simulink model "Attitude_Control_Model_ECX_Flat22L_4Axis"  (R2024b)
settings: Solver=VariableStepAuto  StartTime=0.0  StopTime=10.0  RelTol=1e-3
libraries: slpidlib x7, simulink_extras x2, aerolibutil x2, matrix_library x1
settings Model: Creator=LEGION  LastModifiedBy=LEGION

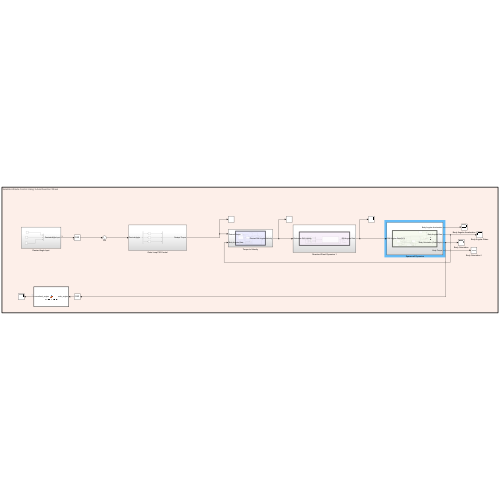
[thumbnail: Simulink's stored preview of the top-level diagram]
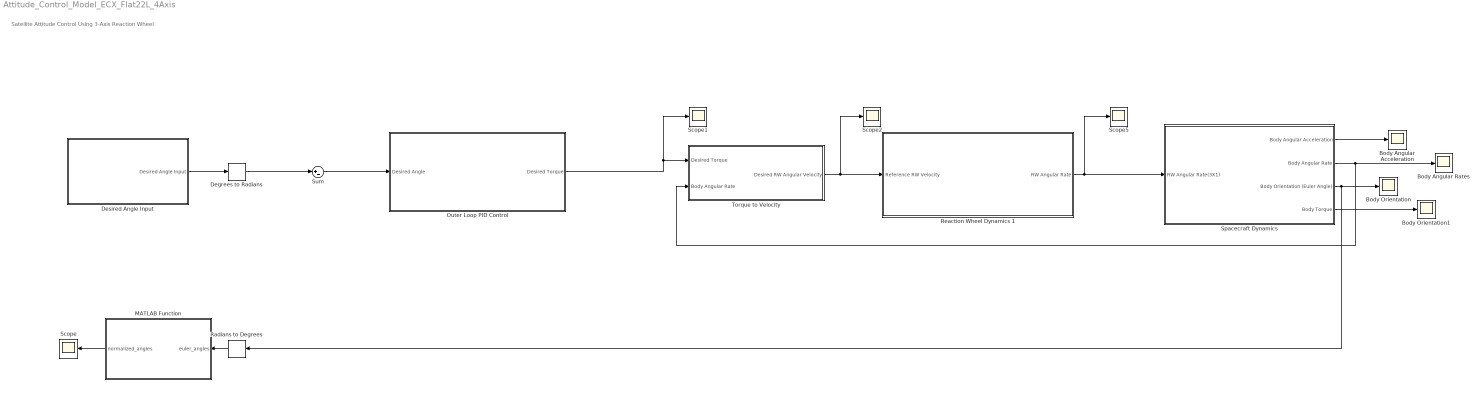
== system Attitude_Control_Model_ECX_Flat22L_4Axis ==
  note: Satellite Attitude Control Using 3-Axis Reaction Wheel
  Body Angular Acceleration : Scope
  Body Angular Rates : Scope
  Body Orientation : Scope
  Body Orientation1 : Scope
  Degrees to Radians : simulink_extras/Transformations/Degrees to Radians
  Desired Angle Input : Subsystem
  MATLAB Function : MATLAB Function  TreatAsAtomicUnit=on
  Outer Loop PID Control : Subsystem
  Radians to Degrees : simulink_extras/Transformations/Radians to Degrees
  Reaction Wheel Dynamics 1 : Subsystem
  Scope{,1..2,5} (4 alike) : Scope
  Spacecraft Dynamics : Subsystem
  Sum : Sum  Inputs=|+-
  Torque to Velocity : Subsystem
  wires:
  Outer Loop PID Control/1(Desired Torque) -> Scope1/1, Torque to Velocity/1(Desired Torque)
  Sum/1 -> Outer Loop PID Control/1(Desired Angle)
  Degrees to Radians/1 -> Sum/1
  Desired Angle Input/1(Desired Angle Input) -> Degrees to Radians/1
  Reaction Wheel Dynamics 1/1(RW Angular Rate) -> Spacecraft Dynamics/1(RW Angular Rate(3X1)), Scope5/1
  Radians to Degrees/1 -> MATLAB Function/1(euler_angles)
  Torque to Velocity/1(Desired RW Angular Velocity) -> Reaction Wheel Dynamics 1/1(Reference RW Velocity), Scope2/1
  MATLAB Function/1(normalized_angles) -> Scope/1
  Spacecraft Dynamics/1(Body Angular Acceleration) -> Body Angular Acceleration/1
  Spacecraft Dynamics/2(Body Angular Rate) -> Torque to Velocity/2(Body Angular Rate), Body Angular Rates/1
  Spacecraft Dynamics/3(Body Orientation (Euler Angle)) -> Radians to Degrees/1, Body Orientation/1
  Spacecraft Dynamics/4(Body Torque) -> Body Orientation1/1

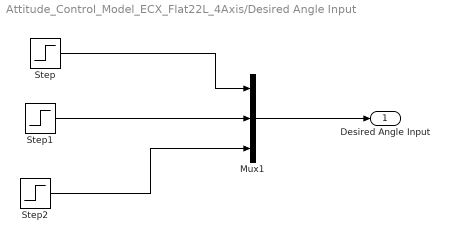
== system Attitude_Control_Model_ECX_Flat22L_4Axis/Desired Angle Input ==
  Mux1 : Mux  Inputs=3
  Step : Step  Time=0.1  After=270  SampleTime=0  VectorParams1D=off
  Step1 : Step  Time=0.1  After=90  SampleTime=0  VectorParams1D=off
  Step2 : Step  Time=0.1  After=90  SampleTime=0  VectorParams1D=off
  Desired Angle Input : Outport
  wires:
  Mux1/1 -> Desired Angle Input/1
  Step1/1 -> Mux1/2
  Step/1 -> Mux1/1
  Step2/1 -> Mux1/3

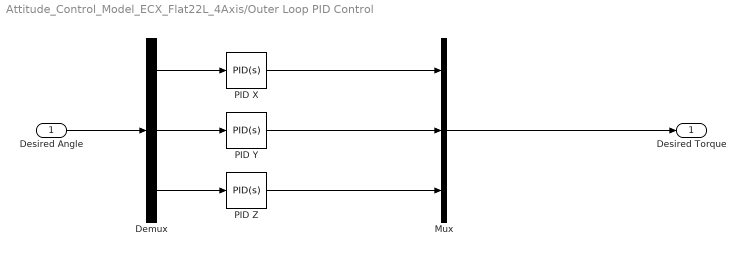
== system Attitude_Control_Model_ECX_Flat22L_4Axis/Outer Loop PID Control ==
  Desired Angle : Inport
  Demux : Demux  Outputs=3
  Mux : Mux  Inputs=3
  PID X : slpidlib/PID Controller  Controller=PID  Form=Parallel  TimeDomain=Continuous-time  UseExternalTs=off  SampleTime=-1  IntegratorMethod=Forward Euler  FilterMethod=Forward Euler  ControllerParametersSource=internal  P=0.8  I=0.007  UseKiTs=off  D=0.5  UseExternalDerivativeSource=off  N=100  UseFilter=on  TunerSelectOption=Transfer Function Based (PID Tuner App)  InitialConditionSource=internal  InitialConditionForIntegrator=0  InitialConditionForFilter=0  DifferentiatorICPrevScaledInput=0  ExternalReset=none  TrackingMode=off  Kt=1  LimitOutput=off  SatLimitsSource=internal  UpperSaturationLimit=inf  LowerSaturationLimit=-inf  LinearizeAsGain=on  AntiWindupMode=none  Kb=1  LimitIntegrator=off  UpperIntegratorSaturationLimit=inf  LowerIntegratorSaturationLimit=-inf  POutMin=[]  POutMax=[]  IOutMin=[]  IOutMax=[]  DOutMin=[]  DOutMax=[]  NOutMin=[]  NOutMax=[]  SumOutMin=[]  SumOutMax=[]  SaturationOutMin=[]  SaturationOutMax=[]  PParamMin=[]  PParamMax=[]  IParamMin=[]  IParamMax=[]  DParamMin=[]  DParamMax=[]  NParamMin=[]  NParamMax=[]  KbParamMin=[]  KbParamMax=[]  KtParamMin=[]  KtParamMax=[]  KbOutMin=[]  KbOutMax=[]  KtOutMin=[]  KtOutMax=[]  IntegratorOutMin=[]  IntegratorOutMax=[]  FilterOutMin=[]  FilterOutMax=[]  SumI1OutMin=[]  SumI1OutMax=[]  SumI2OutMin=[]  SumI2OutMax=[]  SumI3OutMin=[]  SumI3OutMax=[]  SumI4OutMin=[]  SumI4OutMax=[]  SumDOutMin=[]  SumDOutMax=[]  DifferentiatorOutMin=[]  DifferentiatorOutMax=[]  FilterDiffOutCoefMin=[]  FilterDiffOutCoefMax=[]  ReciprocalOutMin=[]  ReciprocalOutMax=[]  SumDenOutMin=[]  SumDenOutMax=[]  SumNumOutMin=[]  SumNumOutMax=[]  DivideOutMin=[]  DivideOutMax=[]  UdiffTsProdOutMin=[]  UdiffTsProdOutMax=[]  NTsProdOutMin=[]  NTsProdOutMax=[]  UintegralTsProdOutMin=[]  UintegralTsProdOutMax=[]  UngainTsProdOutMin=[]  UngainTsProdOutMax=[]  ClampingZeroOutDataTypeStr=Inherit: Inherit via back propagation  ClampingZeroOutMin=[]  ClampingZeroOutMax=[]  FilterDenConstantOutDataTypeStr=Inherit: Inherit via back propagation  FilterDenConstantOutMin=[]  FilterDenConstantOutMax=[]  PCopyOutDataTypeStr=Inherit: Inherit via back propagation  PCopyOutMin=[]  PCopyOutMax=[]  NCopyOutDataTypeStr=Inherit: Inherit via back propagation  NCopyOutMin=[]  NCopyOutMax=[]  IntegratorContinuousStateAttributes=''  IntegratorStateMustResolveToSignalObject=off  IntegratorRTWStateStorageClass=Auto  FilterContinuousStateAttributes=''  FilterStateMustResolveToSignalObject=off  FilterRTWStateStorageClass=Auto  ParallelPVariant=InternalParameters  IdealPVariant=Disabled  IVariant=InternalParameters  DVariant=InternalParameters  IntegratorVariant=Continuous  SatVariant=Disabled  AWVariant=Passthrough  PCopyVariant=Disabled  TRVariant=Disabled  FdbkBlocksVariant=Forward  IdealPFdbkVariant=Disabled  SatFdbkVariant=Disabled  DerivativeFilterVariant=ContFilter  NVariant=InternalParameters  NCopyVariant=Disabled  FilterICVariant=InternalICsFilter  IntegratorICVariant=InternalICs  ExternalResetVariant=Disabled  TRSumVariant=Passthrough  SumFdbkVariant=Disabled  SumVariant=Sum_PID  TsampFilterVariant=InternalTs  TsampNgainVariant=Passthrough  TsampIntegralVariant=Disabled_SignalSpec  ExternalSaturationOutDataTypeStr=Inherit: Same as second input  DerivativeSourceVariant=ErrorSignal  PreIntVariant=InternalPreInt
  PID Y : slpidlib/PID Controller  Controller=PID  Form=Parallel  TimeDomain=Continuous-time  UseExternalTs=off  SampleTime=-1  IntegratorMethod=Forward Euler  FilterMethod=Forward Euler  ControllerParametersSource=internal  P=0.5  I=0.06  UseKiTs=off  D=0.1  UseExternalDerivativeSource=off  N=100  UseFilter=on  TunerSelectOption=Transfer Function Based (PID Tuner App)  InitialConditionSource=internal  InitialConditionForIntegrator=0  InitialConditionForFilter=0  DifferentiatorICPrevScaledInput=0  ExternalReset=none  TrackingMode=off  Kt=1  LimitOutput=off  SatLimitsSource=internal  UpperSaturationLimit=inf  LowerSaturationLimit=-inf  LinearizeAsGain=on  AntiWindupMode=none  Kb=1  LimitIntegrator=off  UpperIntegratorSaturationLimit=inf  LowerIntegratorSaturationLimit=-inf  POutMin=[]  POutMax=[]  IOutMin=[]  IOutMax=[]  DOutMin=[]  DOutMax=[]  NOutMin=[]  NOutMax=[]  SumOutMin=[]  SumOutMax=[]  SaturationOutMin=[]  SaturationOutMax=[]  PParamMin=[]  PParamMax=[]  IParamMin=[]  IParamMax=[]  DParamMin=[]  DParamMax=[]  NParamMin=[]  NParamMax=[]  KbParamMin=[]  KbParamMax=[]  KtParamMin=[]  KtParamMax=[]  KbOutMin=[]  KbOutMax=[]  KtOutMin=[]  KtOutMax=[]  IntegratorOutMin=[]  IntegratorOutMax=[]  FilterOutMin=[]  FilterOutMax=[]  SumI1OutMin=[]  SumI1OutMax=[]  SumI2OutMin=[]  SumI2OutMax=[]  SumI3OutMin=[]  SumI3OutMax=[]  SumI4OutMin=[]  SumI4OutMax=[]  SumDOutMin=[]  SumDOutMax=[]  DifferentiatorOutMin=[]  DifferentiatorOutMax=[]  FilterDiffOutCoefMin=[]  FilterDiffOutCoefMax=[]  ReciprocalOutMin=[]  ReciprocalOutMax=[]  SumDenOutMin=[]  SumDenOutMax=[]  SumNumOutMin=[]  SumNumOutMax=[]  DivideOutMin=[]  DivideOutMax=[]  UdiffTsProdOutMin=[]  UdiffTsProdOutMax=[]  NTsProdOutMin=[]  NTsProdOutMax=[]  UintegralTsProdOutMin=[]  UintegralTsProdOutMax=[]  UngainTsProdOutMin=[]  UngainTsProdOutMax=[]  ClampingZeroOutDataTypeStr=Inherit: Inherit via back propagation  ClampingZeroOutMin=[]  ClampingZeroOutMax=[]  FilterDenConstantOutDataTypeStr=Inherit: Inherit via back propagation  FilterDenConstantOutMin=[]  FilterDenConstantOutMax=[]  PCopyOutDataTypeStr=Inherit: Inherit via back propagation  PCopyOutMin=[]  PCopyOutMax=[]  NCopyOutDataTypeStr=Inherit: Inherit via back propagation  NCopyOutMin=[]  NCopyOutMax=[]  IntegratorContinuousStateAttributes=''  IntegratorStateMustResolveToSignalObject=off  IntegratorRTWStateStorageClass=Auto  FilterContinuousStateAttributes=''  FilterStateMustResolveToSignalObject=off  FilterRTWStateStorageClass=Auto  ParallelPVariant=InternalParameters  IdealPVariant=Disabled  IVariant=InternalParameters  DVariant=InternalParameters  IntegratorVariant=Continuous  SatVariant=Disabled  AWVariant=Passthrough  PCopyVariant=Disabled  TRVariant=Disabled  FdbkBlocksVariant=Forward  IdealPFdbkVariant=Disabled  SatFdbkVariant=Disabled  DerivativeFilterVariant=ContFilter  NVariant=InternalParameters  NCopyVariant=Disabled  FilterICVariant=InternalICsFilter  IntegratorICVariant=InternalICs  ExternalResetVariant=Disabled  TRSumVariant=Passthrough  SumFdbkVariant=Disabled  SumVariant=Sum_PID  TsampFilterVariant=InternalTs  TsampNgainVariant=Passthrough  TsampIntegralVariant=Disabled_SignalSpec  ExternalSaturationOutDataTypeStr=Inherit: Same as second input  DerivativeSourceVariant=ErrorSignal  PreIntVariant=InternalPreInt
  PID Z : slpidlib/PID Controller  Controller=PID  Form=Parallel  TimeDomain=Continuous-time  UseExternalTs=off  SampleTime=-1  IntegratorMethod=Forward Euler  FilterMethod=Forward Euler  ControllerParametersSource=internal  P=0.8  I=0.0005  UseKiTs=off  D=1.5  UseExternalDerivativeSource=off  N=100  UseFilter=on  TunerSelectOption=Transfer Function Based (PID Tuner App)  InitialConditionSource=internal  InitialConditionForIntegrator=0  InitialConditionForFilter=0  DifferentiatorICPrevScaledInput=0  ExternalReset=none  TrackingMode=off  Kt=1  LimitOutput=off  SatLimitsSource=internal  UpperSaturationLimit=inf  LowerSaturationLimit=-inf  LinearizeAsGain=on  AntiWindupMode=none  Kb=1  LimitIntegrator=off  UpperIntegratorSaturationLimit=inf  LowerIntegratorSaturationLimit=-inf  POutMin=[]  POutMax=[]  IOutMin=[]  IOutMax=[]  DOutMin=[]  DOutMax=[]  NOutMin=[]  NOutMax=[]  SumOutMin=[]  SumOutMax=[]  SaturationOutMin=[]  SaturationOutMax=[]  PParamMin=[]  PParamMax=[]  IParamMin=[]  IParamMax=[]  DParamMin=[]  DParamMax=[]  NParamMin=[]  NParamMax=[]  KbParamMin=[]  KbParamMax=[]  KtParamMin=[]  KtParamMax=[]  KbOutMin=[]  KbOutMax=[]  KtOutMin=[]  KtOutMax=[]  IntegratorOutMin=[]  IntegratorOutMax=[]  FilterOutMin=[]  FilterOutMax=[]  SumI1OutMin=[]  SumI1OutMax=[]  SumI2OutMin=[]  SumI2OutMax=[]  SumI3OutMin=[]  SumI3OutMax=[]  SumI4OutMin=[]  SumI4OutMax=[]  SumDOutMin=[]  SumDOutMax=[]  DifferentiatorOutMin=[]  DifferentiatorOutMax=[]  FilterDiffOutCoefMin=[]  FilterDiffOutCoefMax=[]  ReciprocalOutMin=[]  ReciprocalOutMax=[]  SumDenOutMin=[]  SumDenOutMax=[]  SumNumOutMin=[]  SumNumOutMax=[]  DivideOutMin=[]  DivideOutMax=[]  UdiffTsProdOutMin=[]  UdiffTsProdOutMax=[]  NTsProdOutMin=[]  NTsProdOutMax=[]  UintegralTsProdOutMin=[]  UintegralTsProdOutMax=[]  UngainTsProdOutMin=[]  UngainTsProdOutMax=[]  ClampingZeroOutDataTypeStr=Inherit: Inherit via back propagation  ClampingZeroOutMin=[]  ClampingZeroOutMax=[]  FilterDenConstantOutDataTypeStr=Inherit: Inherit via back propagation  FilterDenConstantOutMin=[]  FilterDenConstantOutMax=[]  PCopyOutDataTypeStr=Inherit: Inherit via back propagation  PCopyOutMin=[]  PCopyOutMax=[]  NCopyOutDataTypeStr=Inherit: Inherit via back propagation  NCopyOutMin=[]  NCopyOutMax=[]  IntegratorContinuousStateAttributes=''  IntegratorStateMustResolveToSignalObject=off  IntegratorRTWStateStorageClass=Auto  FilterContinuousStateAttributes=''  FilterStateMustResolveToSignalObject=off  FilterRTWStateStorageClass=Auto  ParallelPVariant=InternalParameters  IdealPVariant=Disabled  IVariant=InternalParameters  DVariant=InternalParameters  IntegratorVariant=Continuous  SatVariant=Disabled  AWVariant=Passthrough  PCopyVariant=Disabled  TRVariant=Disabled  FdbkBlocksVariant=Forward  IdealPFdbkVariant=Disabled  SatFdbkVariant=Disabled  DerivativeFilterVariant=ContFilter  NVariant=InternalParameters  NCopyVariant=Disabled  FilterICVariant=InternalICsFilter  IntegratorICVariant=InternalICs  ExternalResetVariant=Disabled  TRSumVariant=Passthrough  SumFdbkVariant=Disabled  SumVariant=Sum_PID  TsampFilterVariant=InternalTs  TsampNgainVariant=Passthrough  TsampIntegralVariant=Disabled_SignalSpec  ExternalSaturationOutDataTypeStr=Inherit: Same as second input  DerivativeSourceVariant=ErrorSignal  PreIntVariant=InternalPreInt
  Desired Torque : Outport
  wires:
  PID X/1 -> Mux/1
  Demux/1 -> PID X/1
  PID Z/1 -> Mux/3
  Mux/1 -> Desired Torque/1
  Demux/2 -> PID Y/1
  Demux/3 -> PID Z/1
  PID Y/1 -> Mux/2
  Desired Angle/1 -> Demux/1

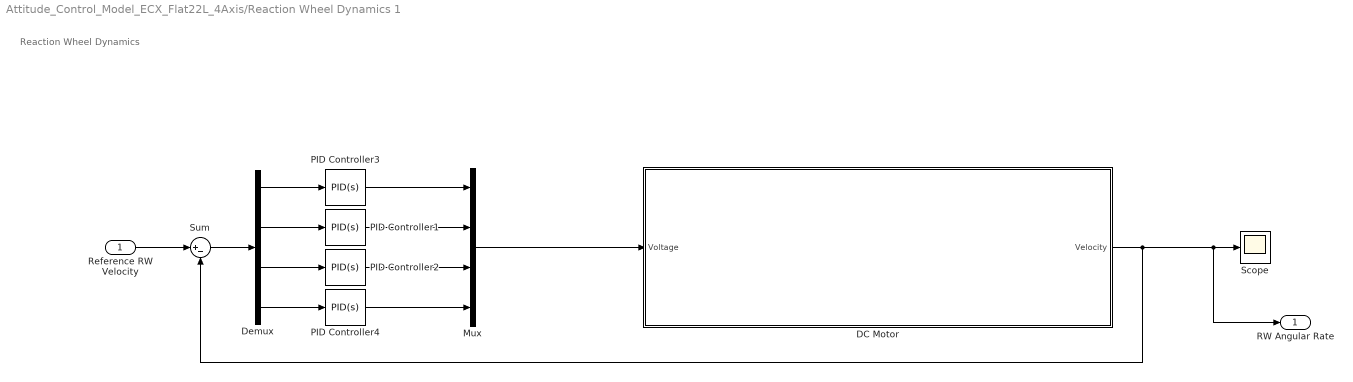
== system Attitude_Control_Model_ECX_Flat22L_4Axis/Reaction Wheel Dynamics 1 ==
  note: Reaction Wheel Dynamics
  Reference RW Velocity : Inport
  "DC Motor " : Subsystem
  Demux : Demux
  Mux : Mux
  PID Controller{1..4} (4 alike) : slpidlib/PID Controller  Controller=PID  Form=Parallel  TimeDomain=Continuous-time  UseExternalTs=off  SampleTime=-1  IntegratorMethod=Forward Euler  FilterMethod=Forward Euler  ControllerParametersSource=internal  P=0.5  I=0.005  UseKiTs=off  D=0.08  UseExternalDerivativeSource=off  N=100  UseFilter=on  TunerSelectOption=Transfer Function Based (PID Tuner App)  InitialConditionSource=internal  InitialConditionForIntegrator=0  InitialConditionForFilter=0  DifferentiatorICPrevScaledInput=0  ExternalReset=none  TrackingMode=off  Kt=1  LimitOutput=off  SatLimitsSource=internal  UpperSaturationLimit=inf  LowerSaturationLimit=-inf  LinearizeAsGain=on  AntiWindupMode=none  Kb=1  LimitIntegrator=off  UpperIntegratorSaturationLimit=inf  LowerIntegratorSaturationLimit=-inf  POutMin=[]  POutMax=[]  IOutMin=[]  IOutMax=[]  DOutMin=[]  DOutMax=[]  NOutMin=[]  NOutMax=[]  SumOutMin=[]  SumOutMax=[]  SaturationOutMin=[]  SaturationOutMax=[]  PParamMin=[]  PParamMax=[]  IParamMin=[]  IParamMax=[]  DParamMin=[]  DParamMax=[]  NParamMin=[]  NParamMax=[]  KbParamMin=[]  KbParamMax=[]  KtParamMin=[]  KtParamMax=[]  KbOutMin=[]  KbOutMax=[]  KtOutMin=[]  KtOutMax=[]  IntegratorOutMin=[]  IntegratorOutMax=[]  FilterOutMin=[]  FilterOutMax=[]  SumI1OutMin=[]  SumI1OutMax=[]  SumI2OutMin=[]  SumI2OutMax=[]  SumI3OutMin=[]  SumI3OutMax=[]  SumI4OutMin=[]  SumI4OutMax=[]  SumDOutMin=[]  SumDOutMax=[]  DifferentiatorOutMin=[]  DifferentiatorOutMax=[]  FilterDiffOutCoefMin=[]  FilterDiffOutCoefMax=[]  ReciprocalOutMin=[]  ReciprocalOutMax=[]  SumDenOutMin=[]  SumDenOutMax=[]  SumNumOutMin=[]  SumNumOutMax=[]  DivideOutMin=[]  DivideOutMax=[]  UdiffTsProdOutMin=[]  UdiffTsProdOutMax=[]  NTsProdOutMin=[]  NTsProdOutMax=[]  UintegralTsProdOutMin=[]  UintegralTsProdOutMax=[]  UngainTsProdOutMin=[]  UngainTsProdOutMax=[]  ClampingZeroOutDataTypeStr=Inherit: Inherit via back propagation  ClampingZeroOutMin=[]  ClampingZeroOutMax=[]  FilterDenConstantOutDataTypeStr=Inherit: Inherit via back propagation  FilterDenConstantOutMin=[]  FilterDenConstantOutMax=[]  PCopyOutDataTypeStr=Inherit: Inherit via back propagation  PCopyOutMin=[]  PCopyOutMax=[]  NCopyOutDataTypeStr=Inherit: Inherit via back propagation  NCopyOutMin=[]  NCopyOutMax=[]  IntegratorContinuousStateAttributes=''  IntegratorStateMustResolveToSignalObject=off  IntegratorRTWStateStorageClass=Auto  FilterContinuousStateAttributes=''  FilterStateMustResolveToSignalObject=off  FilterRTWStateStorageClass=Auto  ParallelPVariant=InternalParameters  IdealPVariant=Disabled  IVariant=InternalParameters  DVariant=InternalParameters  IntegratorVariant=Continuous  SatVariant=Disabled  AWVariant=Passthrough  PCopyVariant=Disabled  TRVariant=Disabled  FdbkBlocksVariant=Forward  IdealPFdbkVariant=Disabled  SatFdbkVariant=Disabled  DerivativeFilterVariant=ContFilter  NVariant=InternalParameters  NCopyVariant=Disabled  FilterICVariant=InternalICsFilter  IntegratorICVariant=InternalICs  ExternalResetVariant=Disabled  TRSumVariant=Passthrough  SumFdbkVariant=Disabled  SumVariant=Sum_PID  TsampFilterVariant=InternalTs  TsampNgainVariant=Passthrough  TsampIntegralVariant=Disabled_SignalSpec  ExternalSaturationOutDataTypeStr=Inherit: Same as second input  DerivativeSourceVariant=ErrorSignal  PreIntVariant=InternalPreInt
  Scope : Scope
  Sum : Sum  Inputs=|+-
  RW Angular Rate : Outport
  wires:
  "DC Motor "/1(Velocity) -> Sum/2, RW Angular Rate/1, Scope/1
  PID Controller1/1 -> Mux/2
  Demux/2 -> PID Controller1/1
  Demux/1 -> PID Controller3/1
  Demux/3 -> PID Controller2/1
  PID Controller3/1 -> Mux/1
  PID Controller2/1 -> Mux/3
  Mux/1 -> "DC Motor "/1(Voltage)
  Reference RW Velocity/1 -> Sum/1
  Sum/1 -> Demux/1
  Demux/4 -> PID Controller4/1
  PID Controller4/1 -> Mux/4

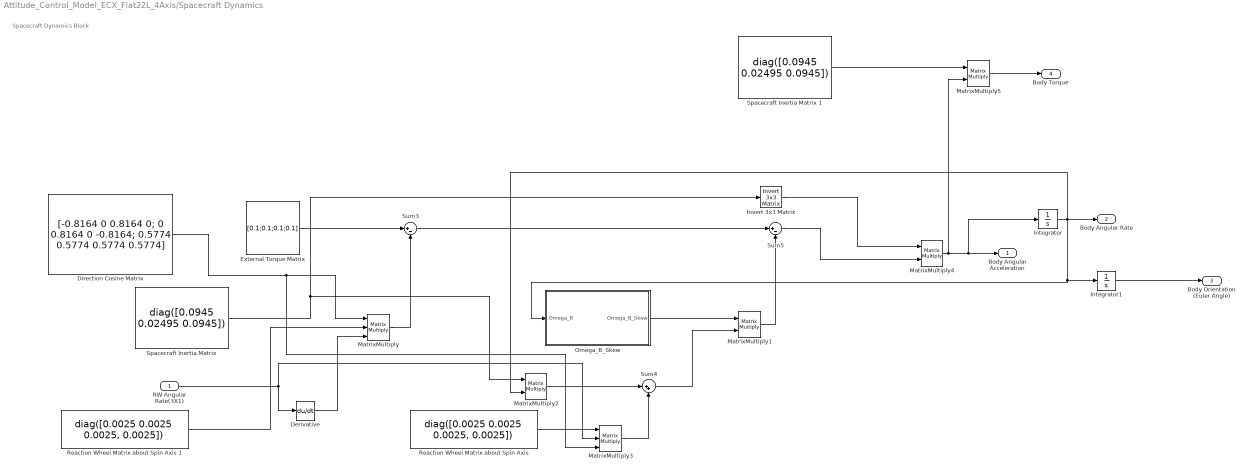
== system Attitude_Control_Model_ECX_Flat22L_4Axis/Spacecraft Dynamics ==
  note: Spacecraft Dynamics Block
  RW Angular Rate(3X1) : Inport
  Derivative : Derivative
  Direction Cosine Matrix : Constant  Value=[-0.8164 0 0.8164 0; 0 0.8164 0 -0.8164; 0.5774 0.5774 0.5774 0.5774]  VectorParams1D=off
  External Torque Matrix : Constant  Value=[0.1;0.1;0.1;0.1]  VectorParams1D=off
  Integrator : Integrator
  Integrator1 : Integrator
  Invert 3x3 Matrix : aerolibutil/Invert  3x3 Matrix
  MatrixMultiply : Product  Inputs=3  Multiplication=Matrix(*)
  MatrixMultiply{1..2,4..5} (4 alike) : Product  Multiplication=Matrix(*)
  MatrixMultiply3 : Product  Inputs=3  Multiplication=Matrix(*)
  Omega_B_Skew : MATLAB Function  TreatAsAtomicUnit=on
  "Reaction Wheel Matrix about Spin Axis " : Constant  Value=diag([0.0025 0.0025 0.0025, 0.0025])  VectorParams1D=off
  Reaction Wheel Matrix about Spin Axis 1 : Constant  Value=diag([0.0025 0.0025 0.0025, 0.0025])  VectorParams1D=off
  "Spacecraft Inertia Matrix " : Constant  Value=diag([0.0945 0.02495 0.0945])  VectorParams1D=off
  Spacecraft Inertia Matrix 1 : Constant  Value=diag([0.0945 0.02495 0.0945])  VectorParams1D=off
  Sum3 : Sum  Inputs=|+-
  Sum4 : Sum  Inputs=|++
  Sum5 : Sum  Inputs=|+-
  Body Angular Acceleration : Outport
  Body Angular Rate : Outport  Port=2
  Body Orientation (Euler Angle) : Outport  Port=3
  Body Torque : Outport  Port=4
  wires:
  "Spacecraft Inertia Matrix "/1 -> MatrixMultiply2/1, Invert 3x3 Matrix/1
  RW Angular Rate(3X1)/1 -> MatrixMultiply3/2, Derivative/1
  Sum4/1 -> MatrixMultiply1/2
  MatrixMultiply2/1 -> Sum4/1
  Integrator/1 -> Omega_B_Skew/1(Omega_B), Integrator1/1, Body Angular Rate/1, MatrixMultiply2/2
  Omega_B_Skew/1(Omega_B_Skew) -> MatrixMultiply1/1
  MatrixMultiply4/1 -> MatrixMultiply5/2, Body Angular Acceleration/1, Integrator/1
  Sum5/1 -> MatrixMultiply4/2
  Invert 3x3 Matrix/1 -> MatrixMultiply4/1
  MatrixMultiply1/1 -> Sum5/2
  "Reaction Wheel Matrix about Spin Axis "/1 -> MatrixMultiply3/1
  Integrator1/1 -> Body Orientation (Euler Angle)/1
  Sum3/1 -> Sum5/1
  Spacecraft Inertia Matrix 1/1 -> MatrixMultiply5/1
  MatrixMultiply3/1 -> Sum4/2
  External Torque Matrix/1 -> Sum3/1
  MatrixMultiply5/1 -> Body Torque/1
  MatrixMultiply/1 -> Sum3/2
  Direction Cosine Matrix/1 -> MatrixMultiply/1, MatrixMultiply3/3
  Reaction Wheel Matrix about Spin Axis 1/1 -> MatrixMultiply/2
  Derivative/1 -> MatrixMultiply/3

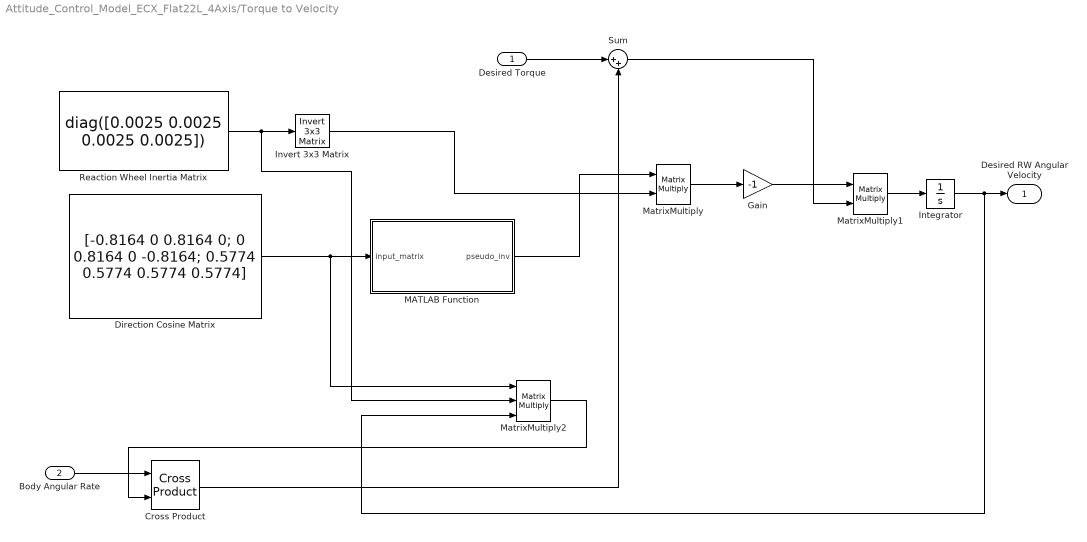
== system Attitude_Control_Model_ECX_Flat22L_4Axis/Torque to Velocity ==
  Desired Torque : Inport
  Body Angular Rate : Inport  Port=2
  Cross Product : matrix_library/Cross Product
  Direction Cosine Matrix : Constant  Value=[-0.8164 0 0.8164 0; 0 0.8164 0 -0.8164; 0.5774 0.5774 0.5774 0.5774]  VectorParams1D=off
  Gain : Gain  Gain=-1
  Integrator : Integrator
  Invert 3x3 Matrix : aerolibutil/Invert  3x3 Matrix
  MATLAB Function : MATLAB Function  TreatAsAtomicUnit=on
  MatrixMultiply : Product  Multiplication=Matrix(*)
  MatrixMultiply1 : Product  Multiplication=Matrix(*)
  MatrixMultiply2 : Product  Inputs=3  Multiplication=Matrix(*)
  Reaction Wheel Inertia Matrix : Constant  Value=diag([0.0025 0.0025 0.0025 0.0025])  VectorParams1D=off
  Sum : Sum  Inputs=|++
  Desired RW Angular Velocity : Outport
  wires:
  Reaction Wheel Inertia Matrix/1 -> MatrixMultiply2/2, Invert 3x3 Matrix/1
  Direction Cosine Matrix/1 -> MatrixMultiply2/1, MATLAB Function/1(input_matrix)
  MATLAB Function/1(pseudo_inv) -> MatrixMultiply/1
  Invert 3x3 Matrix/1 -> MatrixMultiply/2
  MatrixMultiply/1 -> Gain/1
  Desired Torque/1 -> Sum/1
  Body Angular Rate/1 -> Cross Product/1
  MatrixMultiply2/1 -> Cross Product/2
  Cross Product/1 -> Sum/2
  Gain/1 -> MatrixMultiply1/1
  Sum/1 -> MatrixMultiply1/2
  MatrixMultiply1/1 -> Integrator/1
  Integrator/1 -> MatrixMultiply2/3, Desired RW Angular Velocity/1

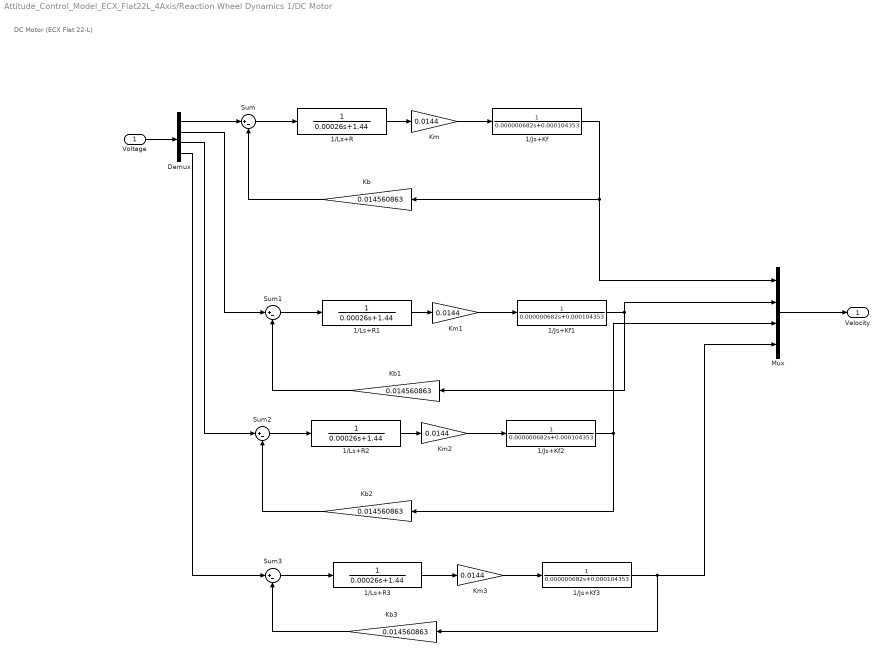
== system Attitude_Control_Model_ECX_Flat22L_4Axis/Reaction Wheel Dynamics 1/DC Motor  ==
  note: DC Motor (ECX Flat 22-L)
  Voltage : Inport
  1/Js+Kf{,1..3} (4 alike) : TransferFcn  Denominator=[0.000000682 0.000104353]
  1/Ls+R{,1..3} (4 alike) : TransferFcn  Denominator=[0.00026 1.44]
  Demux : Demux
  Kb{,1..3} (4 alike) : Gain  Gain=0.014560863
  Km{,1..3} (4 alike) : Gain  Gain=0.0144
  Mux : Mux
  Sum{,1..3} (4 alike) : Sum  Inputs=|+-
  Velocity : Outport
  wires:
  Sum/1 -> 1/Ls+R/1
  1/Ls+R/1 -> Km/1
  Km/1 -> 1/Js+Kf/1
  Kb/1 -> Sum/2
  Voltage/1 -> Demux/1
  Demux/1 -> Sum/1
  Km1/1 -> 1/Js+Kf1/1
  Demux/2 -> Sum1/1
  Kb1/1 -> Sum1/2
  1/Ls+R1/1 -> Km1/1
  1/Js+Kf1/1 -> Kb1/1, Mux/2
  Sum1/1 -> 1/Ls+R1/1
  Km2/1 -> 1/Js+Kf2/1
  Demux/3 -> Sum2/1
  1/Ls+R2/1 -> Km2/1
  1/Js+Kf2/1 -> Kb2/1, Mux/3
  Sum2/1 -> 1/Ls+R2/1
  1/Js+Kf/1 -> Kb/1, Mux/1
  Mux/1 -> Velocity/1
  Kb2/1 -> Sum2/2
  1/Js+Kf3/1 -> Kb3/1, Mux/4
  Km3/1 -> 1/Js+Kf3/1
  1/Ls+R3/1 -> Km3/1
  Sum3/1 -> 1/Ls+R3/1
  Kb3/1 -> Sum3/2
  Demux/4 -> Sum3/1

== matlab function Attitude_Control_Model_ECX_Flat22L_4Axis/Spacecraft Dynamics/Omega_B_Skew ==
  data: Omega_B input; Omega_B_Skew output
function Omega_B_Skew = computeSkewMatrix(Omega_B)
% COMPUTESKEWMATRIX Converts a 3x1 vector into a skew-symmetric matrix.
%
% Inputs:
%   Omega_B - 3x1 vector (angular velocity components in the body frame)
%
% Outputs:
%   Omega_B_Skew - 3x3 skew-symmetric matrix

    % Validate input size
    if size(Omega_B, 1) ~= 3 || size(Omega_B, 2) ~= 1
        error('Input must be a 3x1 vector.');
    end

    % Extract components
    Omega_x = Omega_B(1);
    Omega_y = Omega_B(2);
    Omega_z = Omega_B(3);

    % Create the skew-symmetric matrix
    Omega_B_Skew = [  0       -Omega_z   Omega_y;
                    Omega_z    0        -Omega_x;
                   -Omega_y   Omega_x     0     ];
end

== matlab function Attitude_Control_Model_ECX_Flat22L_4Axis/Torque to Velocity/MATLAB Function ==
  data: input_matrix input; pseudo_inv output
function pseudo_inv = matrix_pseudoinverse(input_matrix)
    % MATRIX_PSEUDOINVERSE Compute the pseudo-inverse of a 3x4 matrix.
    % Usage:
    % pseudo_inv = matrix_pseudoinverse(input_matrix)
    %
    % Input:
    %   input_matrix - A 3x4 matrix.
    %
    % Output:
    %   pseudo_inv - The pseudo-inverse of the input matrix.

    % Validate the input
    [rows, cols] = size(input_matrix);
    if rows ~= 3 || cols ~= 4
        error('Input matrix must be 3x4.');
    end

    % Compute the pseudo-inverse
    pseudo_inv = pinv(input_matrix);
    
    % Display the result
    disp('Pseudo-inverse of the matrix:');
    disp(pseudo_inv);
end

== matlab function Attitude_Control_Model_ECX_Flat22L_4Axis/MATLAB Function ==
  data: euler_angles input; normalized_angles output
function normalized_angles = NormalizedEuler(euler_angles)
% NORMALIZE_EULER_ANGLES Normalizes Euler angles to the range [-180, 180] degrees.
% Input:
%   euler_angles - Nx3 matrix where each row is [x, y, z] Euler angles in degrees
% Output:
%   normalized_angles - Nx3 matrix with normalized Euler angles in the range [-180, 180] degrees

    % Ensure angles are within [-180, 180]
    normalized_angles = mod(euler_angles + 180, 360) - 180;

end
